simulink model "Proposed_method_Yepes2024TTE"  (R2016a)
settings: Solver=FixedStepDiscrete  SolverMode=SingleTasking  StartTime=0.0  StopTime=30  FixedStep=tau_s  RelTol=1e-3
InitFcn:
  | close all
  | clear all
  | clc
  | 
  | tau_s=1e-5;
values from neighbouring files (symbols this model uses):
  backEMF = [0.000292924611226 0.0616187331432 0.124534516601 0.189670464214 0.26371805917 0.336612118136 0.412558888113 0.483874138046 0.547135500724 0.610909554888 0.670449089417 0.731872314514 ... (126 elements, 1x126)]    [backEMF.mat]
undefined symbols (not defined in the file or in its folder): DiscIntNeverNeededParam
libraries: simulink x4, simulink_extras x1, eeGeneralControl x1
settings Model: Creator=Alex  LastModifiedBy=agyepes
settings DataIOCC: ReturnWorkspaceOutputs=on
settings DebuggingCC: SFUnexpectedBacktrackingDiag=error  SFNoUnconditionalDefaultTransitionDiag=error
settings SFSimCC: SimUseLocalCustomCode=on
settings RTWCC: RTWUseLocalCustomCode=on
settings GRTTargetCC: TargetLangStandard=C99 (ISO)
settings ConfigComp: CovMetricSettings=dwe  CovSaveCumulativeToWorkspaceVar=off  CovSaveSingleToWorkspaceVar=off  CovExternalEMLEnable=on

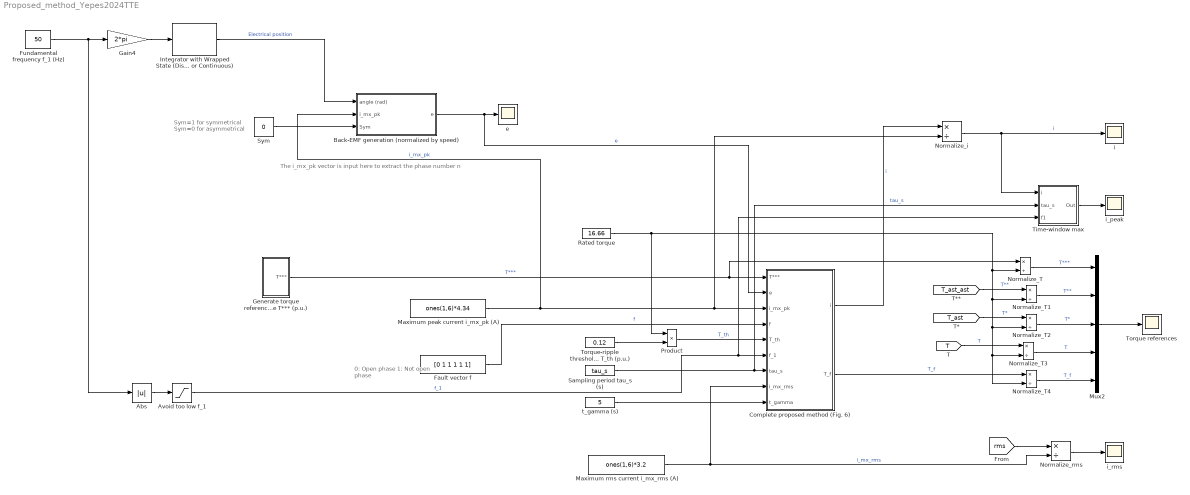
== system Proposed_method_Yepes2024TTE ==
  note: 0: Open phase
      | 1: Not open phase
  note: The i_mx_pk vector is input here to extract the phase number n
  note: Sym=1 for symmetrical
      | Sym=0 for asymmetrical
  Abs : Abs
  Avoid too low f_1 : Saturate  UpperLimit=Inf  LowerLimit=10
  Back-EMF generation (normalized by speed) : Subsystem
      mask init:
      | load('backEMF.mat')
      | load('angle.mat')
  Complete proposed method (Fig. 6) : Subsystem
  Fault vector f : Constant  Value=[0 1 1 1 1 1]
  Fundamental frequency f_1 (Hz) : Constant  Value=50
  Gain4 : Gain  Gain=2*pi
  Generate torque reference T*** (p.u.) : Subsystem
  Integrator with Wrapped State (Discrete or Continuous) : eeGeneralControl/Integrator with Wrapped State (Discrete or Continuous)  OverrideUsingVariant=Discrete  WrappedStateUpperValue=2*pi  WrappedStateLowerValue=0  x0=0  Ts=-1
  Maximum peak current i_mx_pk (A) : Constant  Value=ones(1,6)*4.34
  Maximum rms current i_mx_rms (A) : Constant  Value=ones(1,6)*3.2
  Mux2 : Mux  Inputs=5
  Normalize_T{,1..4} (5 alike) : Product  Inputs=*/
  Normalize_i : Product  Inputs=*/
  Normalize_rms : Product  Inputs=*/
  Product : Product
  Rated torque : Constant  Value=16.66
  Sampling period tau_s (s) : Constant  Value=tau_s
  Sym : Constant  Value=0
  Time-window max : Subsystem
  Torque references : Scope
  Torque-ripple threshold T_th (p.u.) : Constant  Value=0.12
  e : Scope
  i : Scope
  i_peak : Scope
  i_rms : Scope
  t_gamma (s) : Constant  Value=5
  wires:
  Fundamental frequency f_1 (Hz)/1 -> Gain4/1, Abs/1
  Fault vector f/1 -> Complete proposed method (Fig. 6)/4(f)  "f"
  Normalize_i/1 -> Time-window max/1(i), i/1  "i"
  Product/1 -> Complete proposed method (Fig. 6)/5(T_th)  "T_th"
  Sampling period tau_s (s)/1 -> Time-window max/2(tau_s), Complete proposed method (Fig. 6)/7(tau_s)  "tau_s"
  Maximum peak current i_mx_pk (A)/1 -> Back-EMF generation (normalized by speed)/2(i_mx_pk), Normalize_i/2, Complete proposed method (Fig. 6)/3(i_mx_pk)  "i_mx_pk"
  Maximum rms current i_mx_rms (A)/1 -> Normalize_rms/2, Complete proposed method (Fig. 6)/8(i_mx_rms)  "i_mx_rms"
  Normalize_rms/1 -> i_rms/1
  Back-EMF generation (normalized by speed)/1(e) -> Complete proposed method (Fig. 6)/2(e), e/1  "e"
  Gain4/1 -> Integrator with Wrapped State (Discrete or Continuous)/1
  Integrator with Wrapped State (Discrete or Continuous)/1 -> Back-EMF generation (normalized by speed)/1(angle (rad))  "Electrical position"
  Sym/1 -> Back-EMF generation (normalized by speed)/3(Sym)
  Avoid too low f_1/1 -> Time-window max/3(f1), Complete proposed method (Fig. 6)/6(f_1)  "f_1"
  Generate torque reference T*** (p.u.)/1(T***) -> Normalize_T/1, Complete proposed method (Fig. 6)/1(T***)  "T***"
  Complete proposed method (Fig. 6)/1(i) -> Normalize_i/1  "i"
  Time-window max/1(Out) -> i_peak/1
  [rms] -> Normalize_rms/1
  Abs/1 -> Avoid too low f_1/1
  Mux2/1 -> Torque references/1
  Complete proposed method (Fig. 6)/2(T_f) -> Normalize_T4/1  "T_f"
  [T] -> Normalize_T3/1  "T"
  [T_ast] -> Normalize_T2/1  "T*"
  t_gamma (s)/1 -> Complete proposed method (Fig. 6)/9(t_gamma)
  [T_ast_ast] -> Normalize_T1/1  "T**"
  Normalize_T/1 -> Mux2/1  "T***"
  Rated torque/1 -> Product/1, Normalize_T4/2, Normalize_T3/2, Normalize_T2/2, Normalize_T1/2, Normalize_T/2
  Normalize_T1/1 -> Mux2/2  "T**"
  Normalize_T2/1 -> Mux2/3  "T*"
  Normalize_T3/1 -> Mux2/4  "T"
  Normalize_T4/1 -> Mux2/5  "T_f"
  Torque-ripple threshold T_th (p.u.)/1 -> Product/2

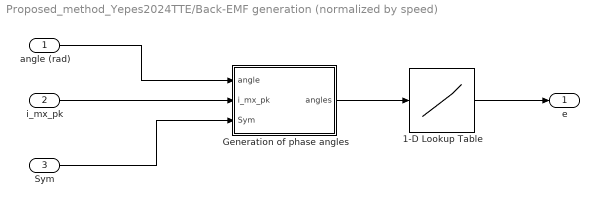
== system Proposed_method_Yepes2024TTE/Back-EMF generation (normalized by speed) ==
  angle (rad) : Inport
  i_mx_pk : Inport  Port=2
  Sym : Inport  Port=3
  1-D Lookup Table : Lookup_n-D  NumberOfTableDimensions=1  BreakpointsForDimension1=angle  Table=backEMF  InternalRulePriority=Speed  RndMeth=Simplest  InputSameDT=on
  Generation of phase angles : MATLAB Function  TreatAsAtomicUnit=on
  e : Outport
  wires:
  1-D Lookup Table/1 -> e/1
  angle (rad)/1 -> Generation of phase angles/1(angle)
  Generation of phase angles/1(angles) -> 1-D Lookup Table/1
  Sym/1 -> Generation of phase angles/3(Sym)
  i_mx_pk/1 -> Generation of phase angles/2(i_mx_pk)

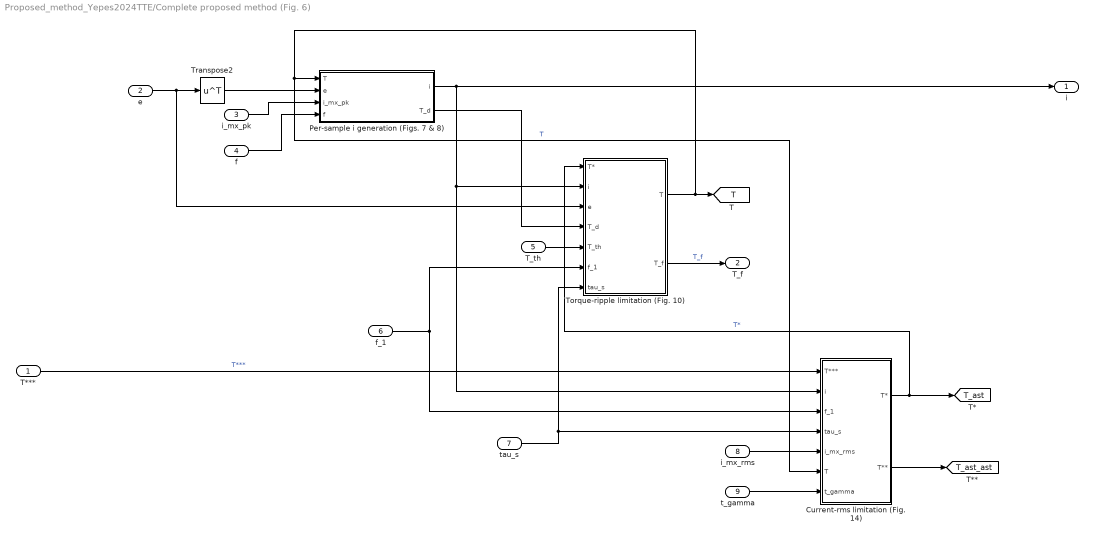
== system Proposed_method_Yepes2024TTE/Complete proposed method (Fig. 6) ==
  T*** : Inport
  e : Inport  Port=2
  i_mx_pk : Inport  Port=3
  f : Inport  Port=4
  T_th : Inport  Port=5
  f_1 : Inport  Port=6
  tau_s : Inport  Port=7
  i_mx_rms : Inport  Port=8
  t_gamma : Inport  Port=9
  Current-rms limitation (Fig. 14) : Subsystem
  Per-sample i generation (Figs. 7 & 8) : MATLAB Function  TreatAsAtomicUnit=on
  Torque-ripple limitation (Fig. 10) : Subsystem
  Transpose2 : Math  Operator=transpose  SaturateOnIntegerOverflow=on
  i : Outport
  T_f : Outport  Port=2
  tag scope: T=global, T_ast=global, T_ast_ast=global
  wires:
  f/1 -> Per-sample i generation (Figs. 7 & 8)/4(f)
  i_mx_pk/1 -> Per-sample i generation (Figs. 7 & 8)/3(i_mx_pk)
  Transpose2/1 -> Per-sample i generation (Figs. 7 & 8)/2(e)
  T***/1 -> Current-rms limitation (Fig. 14)/1(T***)  "T***"
  Current-rms limitation (Fig. 14)/1(T*) -> [T_ast], Torque-ripple limitation (Fig. 10)/1(T*)  "T*"
  i_mx_rms/1 -> Current-rms limitation (Fig. 14)/5(i_mx_rms)
  tau_s/1 -> Torque-ripple limitation (Fig. 10)/7(tau_s), Current-rms limitation (Fig. 14)/4(tau_s)
  Per-sample i generation (Figs. 7 & 8)/1(i) -> Current-rms limitation (Fig. 14)/2(i), Torque-ripple limitation (Fig. 10)/2(i), i/1
  e/1 -> Torque-ripple limitation (Fig. 10)/3(e), Transpose2/1
  f_1/1 -> Current-rms limitation (Fig. 14)/3(f_1), Torque-ripple limitation (Fig. 10)/6(f_1)
  Per-sample i generation (Figs. 7 & 8)/2(T_d) -> Torque-ripple limitation (Fig. 10)/4(T_d)
  T_th/1 -> Torque-ripple limitation (Fig. 10)/5(T_th)
  Torque-ripple limitation (Fig. 10)/1(T) -> [T], Per-sample i generation (Figs. 7 & 8)/1(T), Current-rms limitation (Fig. 14)/6(T)  "T"
  Torque-ripple limitation (Fig. 10)/2(T_f) -> T_f/1  "T_f"
  Current-rms limitation (Fig. 14)/2(T**) -> [T_ast_ast]
  t_gamma/1 -> Current-rms limitation (Fig. 14)/7(t_gamma)

== system Proposed_method_Yepes2024TTE/Generate torque reference T*** (p.u.) ==
  Add : Sum  Inputs=+-
  Ramp1 : simulink/Sources/Ramp  slope=1  start=0  X0=8
  Ramp2 : simulink/Sources/Ramp  slope=3  start=20  X0=0
  Saturation2 : Saturate  UpperLimit=16  LowerLimit=-16
  T*** : Outport
  wires:
  Ramp2/1 -> Add/2
  Ramp1/1 -> Add/1
  Add/1 -> Saturation2/1  "T***"
  Saturation2/1 -> T***/1  "T***"

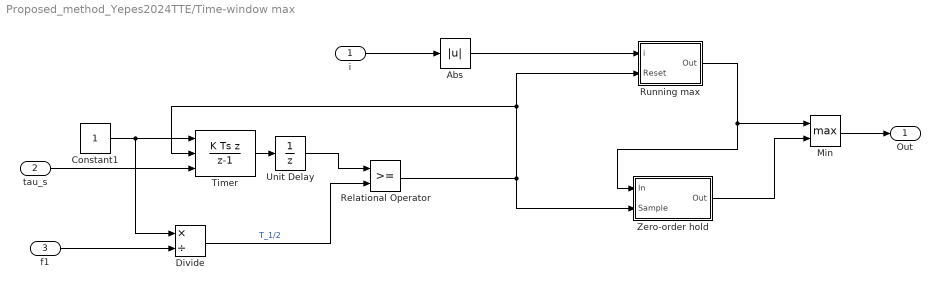
== system Proposed_method_Yepes2024TTE/Time-window max ==
  i : Inport
  tau_s : Inport  Port=2
  f1 : Inport  Port=3
  Abs : Abs
  Constant1 : Constant
  Divide : Product  Inputs=*/
  Min : MinMax  Function=max  Inputs=2
  Relational Operator : RelationalOperator  OutDataTypeStr=boolean
  "Running max " : Subsystem
  Timer : DiscreteIntegrator  IntegratorMethod=Integration: Backward Euler  ExternalReset=rising  InitialConditionSource=external  InitialConditionSetting=State (most efficient)  SampleTime=-1  ICPrevOutput=DiscIntNeverNeededParam  ICPrevScaledInput=DiscIntNeverNeededParam
  Unit Delay : UnitDelay  SampleTime=-1  HasFrameUpgradeWarning=on
  Zero-order hold : Subsystem
  Out : Outport
  wires:
  Min/1 -> Out/1
  Zero-order hold/1(Out) -> Min/2
  "Running max "/1(Out) -> Min/1, Zero-order hold/1(In)
  i/1 -> Abs/1
  Abs/1 -> "Running max "/1(i)
  Divide/1 -> Relational Operator/2  "T_1/2"
  Relational Operator/1 -> Zero-order hold/2(Sample), Timer/2, "Running max "/2(Reset)
  Constant1/1 -> Timer/1, Divide/1
  Unit Delay/1 -> Relational Operator/1
  f1/1 -> Divide/2
  tau_s/1 -> Timer/3
  Timer/1 -> Unit Delay/1

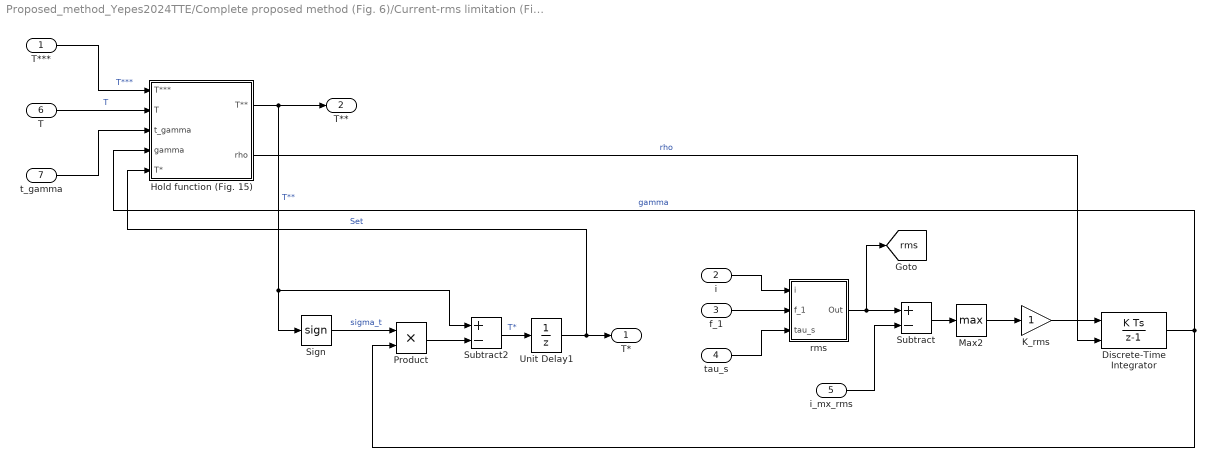
== system Proposed_method_Yepes2024TTE/Complete proposed method (Fig. 6)/Current-rms limitation (Fig. 14) ==
  T*** : Inport
  i : Inport  Port=2
  f_1 : Inport  Port=3
  tau_s : Inport  Port=4
  i_mx_rms : Inport  Port=5
  T : Inport  Port=6
  t_gamma : Inport  Port=7
  Discrete-Time Integrator : DiscreteIntegrator  ExternalReset=rising  InitialConditionSetting=State (most efficient)  SampleTime=-1  LimitOutput=on  LowerSaturationLimit=0  ICPrevOutput=DiscIntNeverNeededParam  ICPrevScaledInput=DiscIntNeverNeededParam
  Hold function (Fig. 15) : Subsystem
  K_rms : Gain
  Max2 : MinMax  Function=max
  Product : Product
  Sign : Signum
  Subtract : Sum  Inputs=+-
  Subtract2 : Sum  Inputs=+-
  Unit Delay1 : UnitDelay  SampleTime=-1  HasFrameUpgradeWarning=on
  rms : Subsystem
  T* : Outport
  T** : Outport  Port=2
  tag scope: rms=global
  wires:
  Subtract/1 -> Max2/1
  Sign/1 -> Product/1  "sigma_t"
  i/1 -> rms/1(i)
  Product/1 -> Subtract2/2
  rms/1(Out) -> [rms], Subtract/1
  Max2/1 -> K_rms/1
  Discrete-Time Integrator/1 -> Product/2, Hold function (Fig. 15)/4(gamma)  "gamma"
  tau_s/1 -> rms/3(tau_s)
  f_1/1 -> rms/2(f_1)
  i_mx_rms/1 -> Subtract/2
  Subtract2/1 -> Unit Delay1/1  "T*"
  Hold function (Fig. 15)/2(rho) -> Discrete-Time Integrator/2  "rho"
  K_rms/1 -> Discrete-Time Integrator/1
  Hold function (Fig. 15)/1(T**) -> Subtract2/1, Sign/1, T**/1  "T**"
  T***/1 -> Hold function (Fig. 15)/1(T***)  "T***"
  T/1 -> Hold function (Fig. 15)/2(T)  "T"
  t_gamma/1 -> Hold function (Fig. 15)/3(t_gamma)
  Unit Delay1/1 -> Hold function (Fig. 15)/5(T*), T*/1  "Set"

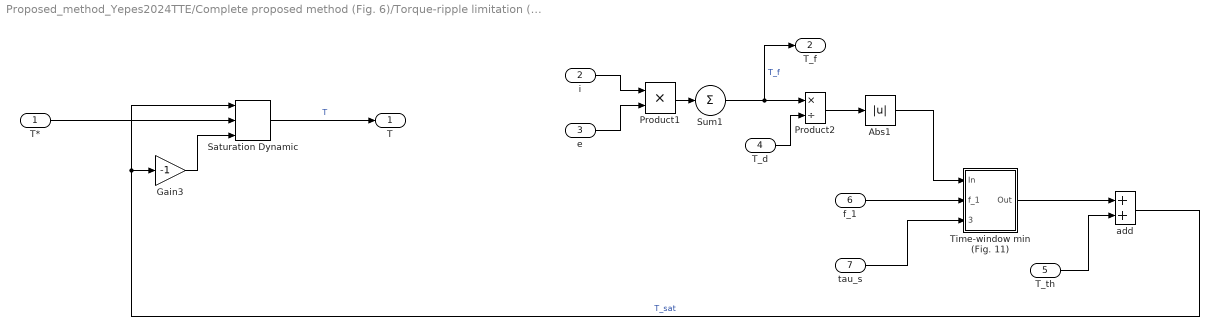
== system Proposed_method_Yepes2024TTE/Complete proposed method (Fig. 6)/Torque-ripple limitation (Fig. 10) ==
  T* : Inport
  i : Inport  Port=2
  e : Inport  Port=3
  T_d : Inport  Port=4
  T_th : Inport  Port=5
  f_1 : Inport  Port=6
  tau_s : Inport  Port=7
  Abs1 : Abs
  Gain3 : Gain  Gain=-1
  Product1 : Product
  Product2 : Product  Inputs=*/
  Saturation Dynamic : simulink/Discontinuities/Saturation Dynamic  OutMin=[]  OutMax=[]  OutDataTypeStr=Inherit: Same as second input  OutDataType=fixdt(1, 16)  OutScaling=2^-10  DoSatur=off
  Sum1 : Sum  Inputs=1
  Time-window min (Fig. 11) : Subsystem
  add : Sum
  T : Outport
  T_f : Outport  Port=2
  wires:
  Product2/1 -> Abs1/1
  Abs1/1 -> Time-window min (Fig. 11)/1(In)
  Product1/1 -> Sum1/1
  Time-window min (Fig. 11)/1(Out) -> add/1
  add/1 -> Gain3/1, Saturation Dynamic/1  "T_sat"
  Gain3/1 -> Saturation Dynamic/3
  Sum1/1 -> T_f/1, Product2/1  "T_f"
  tau_s/1 -> Time-window min (Fig. 11)/3(tau_s)
  T_d/1 -> Product2/2
  e/1 -> Product1/2
  i/1 -> Product1/1
  f_1/1 -> Time-window min (Fig. 11)/2(f_1)
  Saturation Dynamic/1 -> T/1  "T"
  T_th/1 -> add/2
  T*/1 -> Saturation Dynamic/2

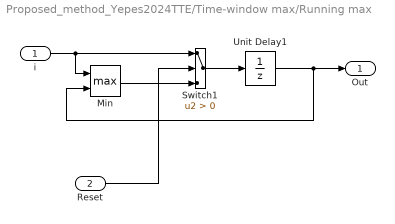
== system Proposed_method_Yepes2024TTE/Time-window max/Running max  ==
  i : Inport
  Reset : Inport  Port=2
  Min : MinMax  Function=max  Inputs=2
  Switch1 : Switch  Criteria=u2 > Threshold
  Unit Delay1 : UnitDelay  SampleTime=-1  HasFrameUpgradeWarning=on
  Out : Outport
  wires:
  Reset/1 -> Switch1/2
  Switch1/1 -> Unit Delay1/1
  i/1 -> Min/1, Switch1/1
  Min/1 -> Switch1/3
  Unit Delay1/1 -> Min/2, Out/1

== system Proposed_method_Yepes2024TTE/Time-window max/Zero-order hold ==
  In : Inport
  Sample : Inport  Port=2
  Switch : Switch  Criteria=u2 > Threshold
  Unit Delay3 : UnitDelay  SampleTime=-1  HasFrameUpgradeWarning=on
  Out : Outport
  wires:
  In/1 -> Switch/1
  Switch/1 -> Unit Delay3/1
  Sample/1 -> Switch/2
  Unit Delay3/1 -> Switch/3, Out/1

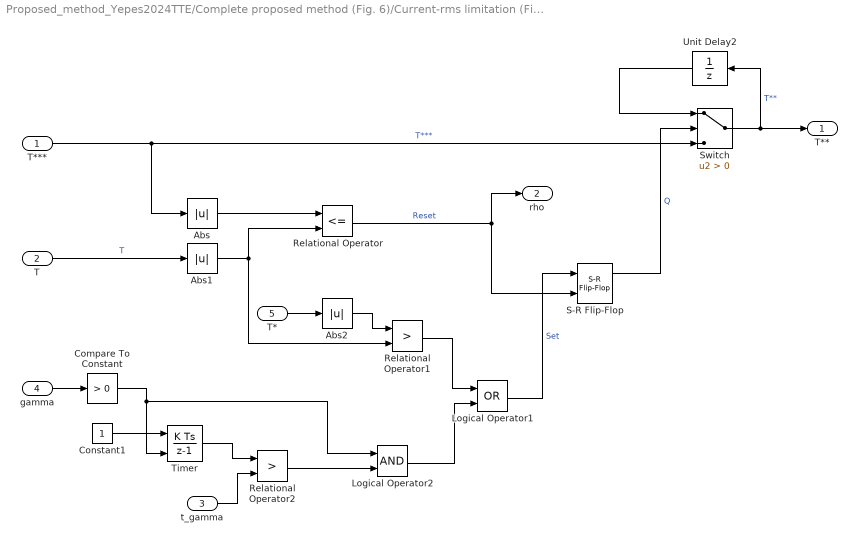
== system Proposed_method_Yepes2024TTE/Complete proposed method (Fig. 6)/Current-rms limitation (Fig. 14)/Hold function (Fig. 15) ==
  T*** : Inport
  T : Inport  Port=2
  t_gamma : Inport  Port=3
  gamma : Inport  Port=4
  T* : Inport  Port=5
  Abs : Abs
  Abs1 : Abs
  Abs2 : Abs
  Compare To Constant : simulink/Logic and Bit Operations/Compare To Constant  relop=>  const=0  OutDataTypeStr=boolean
  Constant1 : Constant
  Logical Operator1 : Logic  Operator=OR  AllPortsSameDT=off  OutDataTypeStr=boolean
  Logical Operator2 : Logic  AllPortsSameDT=off  OutDataTypeStr=boolean
  Relational Operator : RelationalOperator  Operator=<=  OutDataTypeStr=boolean
  Relational Operator1 : RelationalOperator  Operator=>  OutDataTypeStr=boolean
  Relational Operator2 : RelationalOperator  Operator=>  OutDataTypeStr=boolean
  S-R Flip-Flop : simulink_extras/Flip Flops/S-R Flip-Flop  initial_condition=0
  Switch : Switch  Criteria=u2 > Threshold
  Timer : DiscreteIntegrator  ExternalReset=rising  InitialConditionSetting=State (most efficient)  SampleTime=-1  ICPrevOutput=DiscIntNeverNeededParam  ICPrevScaledInput=DiscIntNeverNeededParam
  Unit Delay2 : UnitDelay  SampleTime=-1  HasFrameUpgradeWarning=on
  T** : Outport
  rho : Outport  Port=2
  wires:
  Constant1/1 -> Timer/1
  Switch/1 -> T**/1, Unit Delay2/1  "T**"
  Compare To Constant/1 -> Logical Operator2/1, Timer/2
  Relational Operator/1 -> rho/1, S-R Flip-Flop/2  "Reset"
  Unit Delay2/1 -> Switch/1
  S-R Flip-Flop/1 -> Switch/2  "Q"
  Timer/1 -> Relational Operator2/1
  gamma/1 -> Compare To Constant/1
  Logical Operator1/1 -> S-R Flip-Flop/1  "Set"
  Relational Operator2/1 -> Logical Operator2/2
  T/1 -> Abs1/1  "T"
  Relational Operator1/1 -> Logical Operator1/1
  T***/1 -> Abs/1, Switch/3  "T***"
  Logical Operator2/1 -> Logical Operator1/2
  t_gamma/1 -> Relational Operator2/2
  T*/1 -> Abs2/1
  Abs/1 -> Relational Operator/1
  Abs1/1 -> Relational Operator/2, Relational Operator1/2
  Abs2/1 -> Relational Operator1/1

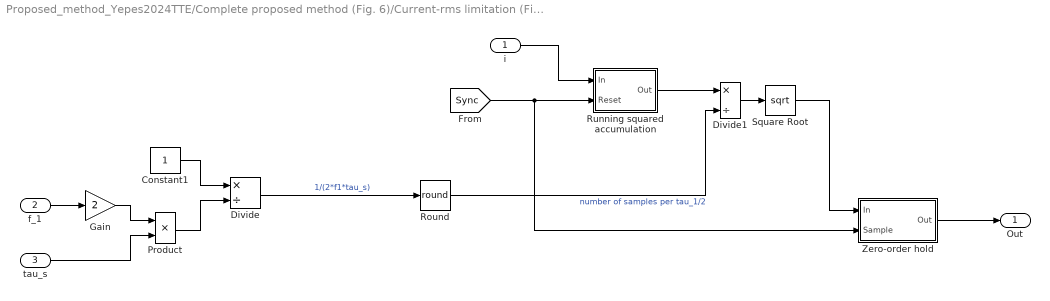
== system Proposed_method_Yepes2024TTE/Complete proposed method (Fig. 6)/Current-rms limitation (Fig. 14)/rms ==
  i : Inport
  f_1 : Inport  Port=2
  tau_s : Inport  Port=3
  Constant1 : Constant
  Divide : Product  Inputs=*/
  Divide1 : Product  Inputs=*/
  Gain : Gain  Gain=2
  Product : Product
  Round : Rounding  Operator=round
  "Running squared accumulation " : Subsystem
  Square Root : Sqrt  SaturateOnIntegerOverflow=on
  Zero-order hold : Subsystem
  Out : Outport
  wires:
  Divide1/1 -> Square Root/1
  [Sync] -> "Running squared accumulation "/2(Reset), Zero-order hold/2(Sample)
  Round/1 -> Divide1/2  "number of samples per tau_1/2"
  Product/1 -> Divide/2
  Divide/1 -> Round/1  "1/(2*f1*tau_s)"
  Square Root/1 -> Zero-order hold/1(In)
  "Running squared accumulation "/1(Out) -> Divide1/1
  Constant1/1 -> Divide/1
  i/1 -> "Running squared accumulation "/1(In)
  tau_s/1 -> Product/2
  f_1/1 -> Gain/1
  Zero-order hold/1(Out) -> Out/1
  Gain/1 -> Product/1

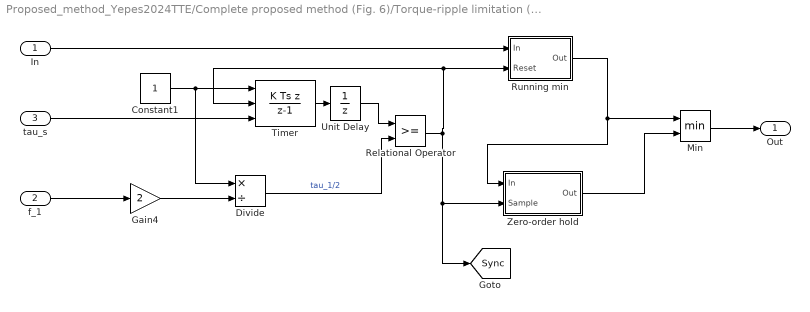
== system Proposed_method_Yepes2024TTE/Complete proposed method (Fig. 6)/Torque-ripple limitation (Fig. 10)/Time-window min (Fig. 11) ==
  In : Inport
  f_1 : Inport  Port=2
  tau_s : Inport  Port=3
  Constant1 : Constant
  Divide : Product  Inputs=*/
  Gain4 : Gain  Gain=2
  Min : MinMax  Inputs=2
  Relational Operator : RelationalOperator  OutDataTypeStr=boolean
  "Running min " : Subsystem
  Timer : DiscreteIntegrator  IntegratorMethod=Integration: Backward Euler  ExternalReset=rising  InitialConditionSource=external  InitialConditionSetting=State (most efficient)  SampleTime=-1  ICPrevOutput=DiscIntNeverNeededParam  ICPrevScaledInput=DiscIntNeverNeededParam
  Unit Delay : UnitDelay  SampleTime=-1  HasFrameUpgradeWarning=on
  Zero-order hold : Subsystem
  Out : Outport
  tag scope: Sync=global
  wires:
  Min/1 -> Out/1
  f_1/1 -> Gain4/1
  Gain4/1 -> Divide/2
  Zero-order hold/1(Out) -> Min/2
  "Running min "/1(Out) -> Min/1, Zero-order hold/1(In)
  Relational Operator/1 -> "Running min "/2(Reset), Timer/2, [Sync], Zero-order hold/2(Sample)
  In/1 -> "Running min "/1(In)
  Divide/1 -> Relational Operator/2  "tau_1/2"
  Constant1/1 -> Timer/1, Divide/1
  Timer/1 -> Unit Delay/1
  Unit Delay/1 -> Relational Operator/1
  tau_s/1 -> Timer/3

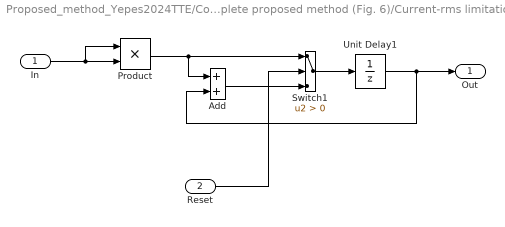
== system Proposed_method_Yepes2024TTE/Complete proposed method (Fig. 6)/Current-rms limitation (Fig. 14)/rms/Running squared accumulation  ==
  In : Inport
  Reset : Inport  Port=2
  Add : Sum
  Product : Product
  Switch1 : Switch  Criteria=u2 > Threshold
  Unit Delay1 : UnitDelay  SampleTime=-1  HasFrameUpgradeWarning=on
  Out : Outport
  wires:
  Reset/1 -> Switch1/2
  Switch1/1 -> Unit Delay1/1
  Add/1 -> Switch1/3
  Unit Delay1/1 -> Add/2, Out/1
  In/1 -> Product/2, Product/1
  Product/1 -> Add/1, Switch1/1

== system Proposed_method_Yepes2024TTE/Complete proposed method (Fig. 6)/Current-rms limitation (Fig. 14)/rms/Zero-order hold ==
  In : Inport
  Sample : Inport  Port=2
  Switch : Switch  Criteria=u2 > Threshold
  Unit Delay3 : UnitDelay  SampleTime=-1  HasFrameUpgradeWarning=on
  Out : Outport
  wires:
  In/1 -> Switch/1
  Switch/1 -> Unit Delay3/1
  Sample/1 -> Switch/2
  Unit Delay3/1 -> Switch/3, Out/1

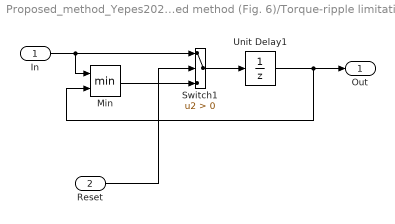
== system Proposed_method_Yepes2024TTE/Complete proposed method (Fig. 6)/Torque-ripple limitation (Fig. 10)/Time-window min (Fig. 11)/Running min  ==
  In : Inport
  Reset : Inport  Port=2
  Min : MinMax  Inputs=2
  Switch1 : Switch  Criteria=u2 > Threshold
  Unit Delay1 : UnitDelay  InitialCondition=Inf  SampleTime=-1  HasFrameUpgradeWarning=on
  Out : Outport
  wires:
  Reset/1 -> Switch1/2
  Switch1/1 -> Unit Delay1/1
  In/1 -> Min/1, Switch1/1
  Min/1 -> Switch1/3
  Unit Delay1/1 -> Min/2, Out/1

== system Proposed_method_Yepes2024TTE/Complete proposed method (Fig. 6)/Torque-ripple limitation (Fig. 10)/Time-window min (Fig. 11)/Zero-order hold ==
  In : Inport
  Sample : Inport  Port=2
  Switch : Switch  Criteria=u2 > Threshold
  Unit Delay3 : UnitDelay  InitialCondition=Inf  SampleTime=-1  HasFrameUpgradeWarning=on
  Out : Outport
  wires:
  In/1 -> Switch/1
  Switch/1 -> Unit Delay3/1
  Sample/1 -> Switch/2
  Unit Delay3/1 -> Switch/3, Out/1

== matlab function Proposed_method_Yepes2024TTE/Complete proposed method (Fig. 6)/Per-sample i generation (Figs. 7 & 8) ==
  data: T input; e input; i output; i_mx_pk input; f input; T_d output
function [i,T_d] = fcn(T,e,i_mx_pk,f)
%Proposed method to compute current references i_ref

n=length(e);%Phase number
f_v=f;f_nv=zeros(n,1);f_nvs=zeros(n,1);%Initially, consider all healthy currents as variables
T_d=0;%Initialize Td

[i_v,i_nv]=compute_inv_iv(T,f_v,f_nv,f_nvs);%Compute optimum i_v
f_v_prime=double(abs(i_v)<i_mx_pk.*f_v);%Check which variable phase currents are below the limit
    
%Iterate until no phase currents exceed the limit or T unfeasible (i.e., i_v contains Inf or Nan, or the number of i_v values below the limit is one or none)
while any(f_v_prime~=f_v) && sum(f_v_prime)>1 && not(any(isinf(i_v))) && not(any(isnan(i_v)))
    f_v=f_v_prime;%Restrict the number of variable currents i_v
    f_nvs=f_nvs+double(not(f_v_prime)).*sign(i_v);%Set signs of new i_nv terms
    f_nv=abs(f_nvs);%Extend the number of non-variable currents i_nv
    [i_v,i_nv]=compute_inv_iv(T,f_v,f_nv,f_nvs);%Compute optimum i_nv and i_v
    f_v_prime=double(abs(i_v)<i_mx_pk.*f_v);%Check which variable phase currents are below the limit
end

%If T cannot be reached while respecting i_mx_pk and (12), maximize T
if sum(f_v_prime)<=1 || any(isinf(i_v)) || any(isnan(i_v))
    T_d=1;
    i_v=zeros(n,1);i_nv=zeros(n,1);%Reset i_v and i_nv
    sigma_T=sign(T);%Identify T sign
    sigma_e=sign(sum(sign(e.*f)));%Identify predominant e sign
    if sigma_e==0%Same number of positive and negative e terms
        i_nv=sigma_T*i_mx_pk.*sign(e.*f);
    else
        kappa_plus=(sign(e)==sigma_e)&f;%kappa_plus=k indices of e_k with sign equal to sigma_e
        kappa_minus=(sign(e)~=sigma_e)&f;%kappa_minus=k indices of e_k with sign different from sigma_e
        n_kappa_plus=sum(kappa_plus);%Number of kappa_plus indices
        n_kappa_minus=sum(kappa_minus);%Number of kappa_minus indices
        i_nv(kappa_minus)=-sigma_T*sigma_e*i_mx_pk(kappa_minus);%Set to -sigma_T*sigma_e*i^mx_pk the i_k,nv with k=kappa_minus
        [~,kappa_s]=sort(sigma_e*e.*f);%kappa_s=k indices sorted so that sigma_e*e_k*f_k is in ascending order
        for k=1:n_kappa_minus
            i_nv(kappa_s(length(e)+1-k))=sigma_T*sigma_e*i_mx_pk(kappa_s(length(e)+1-k));%Set to sigma_T*sigma_e*i^mx_k,pk the i_k,nv with k=kappa_plus corresponding to the #n_kappa_minus largest |e_k|
        end
        for k=1:floor((n_kappa_plus-n_kappa_minus)/2) %Among the remaining #(kappa_plus-kappa_minus) elements of i_k,nv with k=kappa_plus, set to -sigma_T*sigma_e*i^mx_k,pk and to sigma_T*sigma_e*i^mx_k,pk those corresponding to the #floor(kappa_plus-kappa_minus) lowest and largest |e_k|, respectively
            i_nv(kappa_s(sum(not(f))+n_kappa_minus+k))=-sigma_T*sigma_e*i_mx_pk(kappa_s(sum(not(f))+n_kappa_minus+k));
            i_nv(kappa_s(length(e)+1-n_kappa_minus-k))=sigma_T*sigma_e*i_mx_pk(kappa_s(length(e)+1-n_kappa_minus-k));
        end
    end 
end

i=i_v'+i_nv';%Combine i_v and i_nv in total references

%Function to compute i_nv and i_v for minimum SCL
function [i_v,i_nv]=compute_inv_iv(T_ref,f_v,f_nv,f_nvs)
    i_nv=i_mx_pk.*f_nvs;%Set non-variable currents to the limit
    fve=f_v.*e;fvte=f_v'*e;ff=f_v'*f_v;fvteff=fvte/ff;%Auxiliary variables for (12) and (13)
    fnve=f_nv.*e;fvfnvtiff=f_v*(f_nv'*i_nv/ff);%Auxiliary variables for (12) and (13)
    T_nv=fnve'*i_nv-fve'*fvfnvtiff;%Torque due to i_nv (13)
    num=(fve-fvteff*f_v)*(T_ref-T_nv);%Numerator of first fraction in equation (12)
    den=fve'*e-fvteff*fvte;%Denominator of first fraction in equation (12)
    i_v=num/den-fvfnvtiff;%Calculate variable currents using (12)
end

end

== matlab function Proposed_method_Yepes2024TTE/Back-EMF generation (normalized by speed)/Generation of phase angles ==
  data: angle input; i_mx_pk input; angles output; Sym input
function angles = fcn(angle,i_mx_pk,Sym)

n=length(i_mx_pk);%Extract phase number
angles=zeros(1,n);
if Sym==1 %Symmetrical windings
    for k=1:n
        angles(k) = wrapTo2Pi(angle-(k-1)*2*pi/n);
    end
else %Asymmetrical windings
    k=0;
    for k1=1:3
        for k2=1:n/3
            k=k+1;
            angles(k) = wrapTo2Pi(angle-(k1-1)*2*pi/3-(k2-1)*pi/n);
        end
    end    
end
